simulink library "AtmosphericModel"  (R2024a)
settings: Solver=ode45  StartTime=0.0  StopTime=10.0  RelTol=1e-3  EnableMultiTasking=on
settings Model: Creator=bruno  LastModifiedBy=Caê
settings SolverCC: AlgebraicLoopSolver=TrustRegion
settings DataIOCC: LimitDataPoints=on  ReturnWorkspaceOutputs=off
settings OptimizationCC: LifeSpan=inf
settings DebuggingCC: UnconnectedInputMsg=warning  UnconnectedOutputMsg=warning  UnconnectedLineMsg=warning  AllowSymbolicDim=off  SFUnexpectedBacktrackingDiag=warning  SFNoUnconditionalDefaultTransitionDiag=warning  ArithmeticOperatorsInVariantConditions=warning
settings ModelReferenceCC: EnableRefExpFcnMdlSchedulingChecks=on
settings SFSimCC: SimUseLocalCustomCode=off  CustomCodeUndefinedFunction=UseInterfaceOnly
settings RTWCC: RTWUseLocalCustomCode=off  GPUComputeCapability=3.5
settings CodeAppCC: StateflowObjectComments=on
settings GRTTargetCC: TargetLangStandard=C89/C90 (ANSI)
settings ConfigComp: CovMetricSettings=dw  CovSaveCumulativeToWorkspaceVar=on  CovSaveSingleToWorkspaceVar=on  CovExternalEMLEnable=off

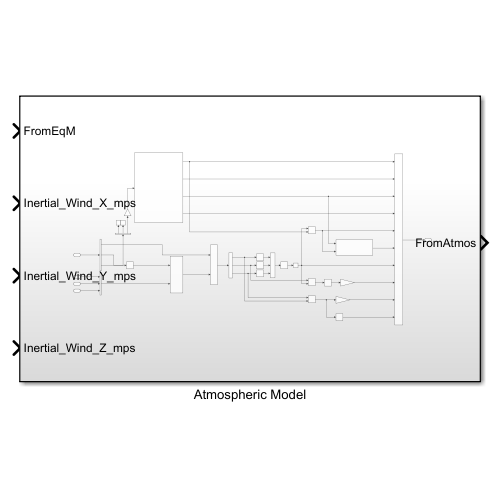
[thumbnail: Simulink's stored preview of the top-level diagram]
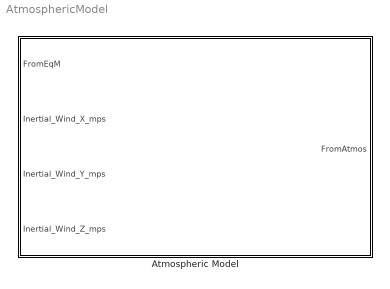
== system AtmosphericModel ==
  Atmospheric Model : Subsystem

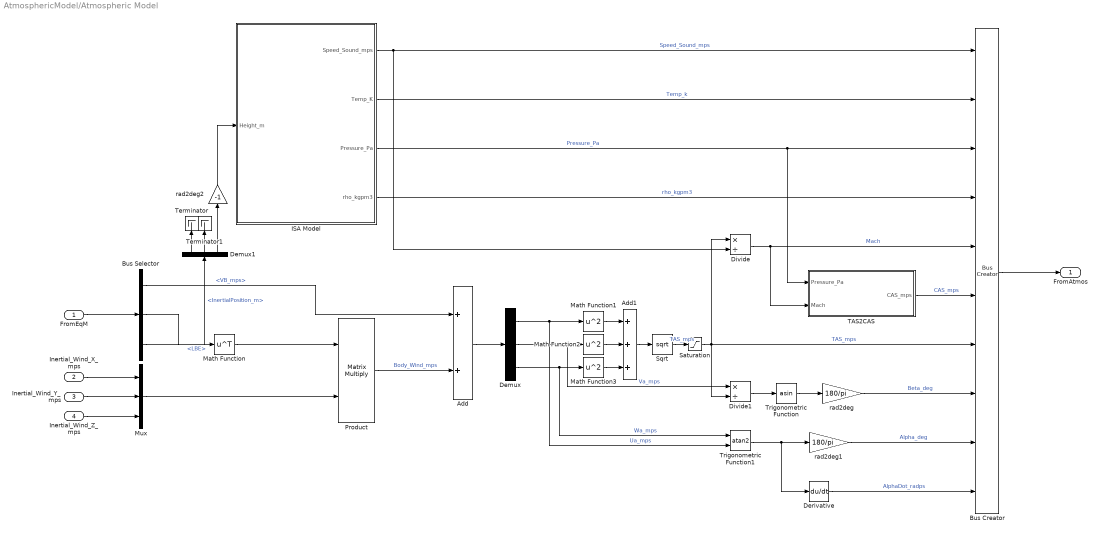
== system AtmosphericModel/Atmospheric Model ==
  FromEqM : Inport
  Inertial_Wind_X_mps : Inport  Port=2
  Inertial_Wind_Y_mps : Inport  Port=3
  Inertial_Wind_Z_mps : Inport  Port=4
  Add : Sum
  Add1 : Sum  Inputs=+++
  Bus Creator : BusCreator  Inputs=10
  Bus Selector : BusSelector  OutputSignals=VB_mps,LBE,InertialPosition_m
  Demux : Demux  Outputs=3
  Demux1 : Demux  Outputs=3
  Derivative : Derivative
  Divide : Product  Inputs=*/
  Divide1 : Product  Inputs=*/
  ISA Model : Subsystem
  Math Function : Math  Operator=transpose  SignedPower=on
  Math Function1 : Math  Operator=square  SignedPower=on
  Math Function2 : Math  Operator=square  SignedPower=on
  Math Function3 : Math  Operator=square  SignedPower=on
  Mux : Mux  Inputs=3
  Product : Product  Multiplication=Matrix(*)
  Saturation : Saturate  UpperLimit=Inf  LowerLimit=0.01
  Sqrt : Sqrt
  TAS2CAS : Subsystem
  Terminator : Terminator
  Terminator1 : Terminator
  Trigonometric Function : Trigonometry  Operator=asin
  Trigonometric Function1 : Trigonometry  Operator=atan2
  rad2deg : Gain  Gain=180/pi
  rad2deg1 : Gain  Gain=180/pi
  rad2deg2 : Gain  Gain=-1
  FromAtmos : Outport
  wires:
  Bus Selector/3 -> Demux1/1  "<InertialPosition_m>"
  Saturation/1 -> Bus Creator/7, Divide1/2, Divide/1  "TAS_mps"
  rad2deg2/1 -> ISA Model/1("Height_m ")
  Demux1/2 -> Terminator1/1
  Demux1/1 -> Terminator/1
  Bus Selector/1 -> Add/1  "<VB_mps>"
  Bus Selector/2 -> Math Function/1  "<LBE>"
  Derivative/1 -> Bus Creator/10  "AlphaDot_radps"
  Trigonometric Function1/1 -> rad2deg1/1, Derivative/1
  Bus Creator/1 -> FromAtmos/1
  rad2deg1/1 -> Bus Creator/9  "Alpha_deg"
  ISA Model/4(rho_kgpm3) -> Bus Creator/4  "rho_kgpm3"
  ISA Model/1(Speed_Sound_mps) -> Divide/2, Bus Creator/1  "Speed_Sound_mps"
  Inertial_Wind_Y_mps/1 -> Mux/2
  ISA Model/2(Temp_K) -> Bus Creator/2  "Temp_k"
  Inertial_Wind_X_mps/1 -> Mux/1
  ISA Model/3(Pressure_Pa) -> Bus Creator/3, TAS2CAS/1(Pressure_Pa)  "Pressure_Pa"
  Divide/1 -> TAS2CAS/2(Mach), Bus Creator/5  "Mach"
  FromEqM/1 -> Bus Selector/1
  Sqrt/1 -> Saturation/1  "TAS_mps"
  Inertial_Wind_Z_mps/1 -> Mux/3
  Math Function/1 -> Product/1
  Mux/1 -> Product/2
  Product/1 -> Add/2  "Body_Wind_mps"
  TAS2CAS/1(CAS_mps) -> Bus Creator/6  "CAS_mps"
  Demux1/3 -> rad2deg2/1
  Add/1 -> Demux/1
  Demux/1 -> Math Function1/1, Trigonometric Function1/2  "Ua_mps"
  Math Function2/1 -> Add1/2
  Trigonometric Function/1 -> rad2deg/1
  Divide1/1 -> Trigonometric Function/1
  Demux/3 -> Math Function3/1, Trigonometric Function1/1  "Wa_mps"
  Demux/2 -> Math Function2/1, Divide1/1  "Va_mps"
  Math Function1/1 -> Add1/1
  Add1/1 -> Sqrt/1
  Math Function3/1 -> Add1/3
  rad2deg/1 -> Bus Creator/8  "Beta_deg"

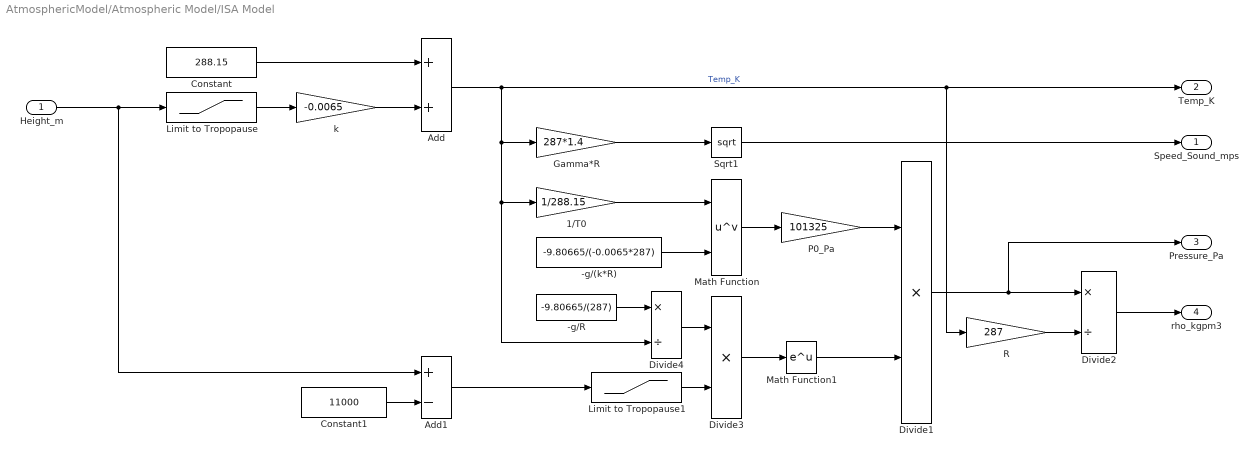
== system AtmosphericModel/Atmospheric Model/ISA Model ==
  "Height_m " : Inport
  -g/(k*R) : Constant  Value=-9.80665/(-0.0065*287)
  -g/R : Constant  Value=-9.80665/(287)
  1/T0 : Gain  Gain=1/288.15
  Add : Sum
  Add1 : Sum  Inputs=+-
  Constant : Constant  Value=288.15
  Constant1 : Constant  Value=11000
  Divide1 : Product  Inputs=**
  Divide2 : Product  Inputs=*/
  Divide3 : Product  Inputs=**
  Divide4 : Product  Inputs=*/
  Gamma*R : Gain  Gain=287*1.4
  Limit to Tropopause : Saturate  UpperLimit=11000  LowerLimit=0
  Limit to Tropopause1 : Saturate  UpperLimit=inf  LowerLimit=0
  Math Function : Math  Operator=pow  SignedPower=on
  Math Function1 : Math  SignedPower=on
  P0_Pa : Gain  Gain=101325
  R : Gain  Gain=287
  Sqrt1 : Sqrt
  k : Gain  Gain=-0.0065
  Speed_Sound_mps : Outport
  Temp_K : Outport  Port=2
  Pressure_Pa : Outport  Port=3
  rho_kgpm3 : Outport  Port=4
  wires:
  Gamma*R/1 -> Sqrt1/1
  Limit to Tropopause/1 -> k/1
  Add/1 -> Divide4/2, 1/T0/1, Gamma*R/1, Temp_K/1, R/1  "Temp_K"
  k/1 -> Add/2
  Constant/1 -> Add/1
  "Height_m "/1 -> Add1/1, Limit to Tropopause/1
  Add1/1 -> Limit to Tropopause1/1
  Limit to Tropopause1/1 -> Divide3/2
  Sqrt1/1 -> Speed_Sound_mps/1
  1/T0/1 -> Math Function/1
  -g/(k*R)/1 -> Math Function/2
  Math Function/1 -> P0_Pa/1
  P0_Pa/1 -> Divide1/1
  Divide1/1 -> Divide2/1, Pressure_Pa/1
  R/1 -> Divide2/2
  Divide2/1 -> rho_kgpm3/1
  Constant1/1 -> Add1/2
  -g/R/1 -> Divide4/1
  Divide4/1 -> Divide3/1
  Divide3/1 -> Math Function1/1
  Math Function1/1 -> Divide1/2

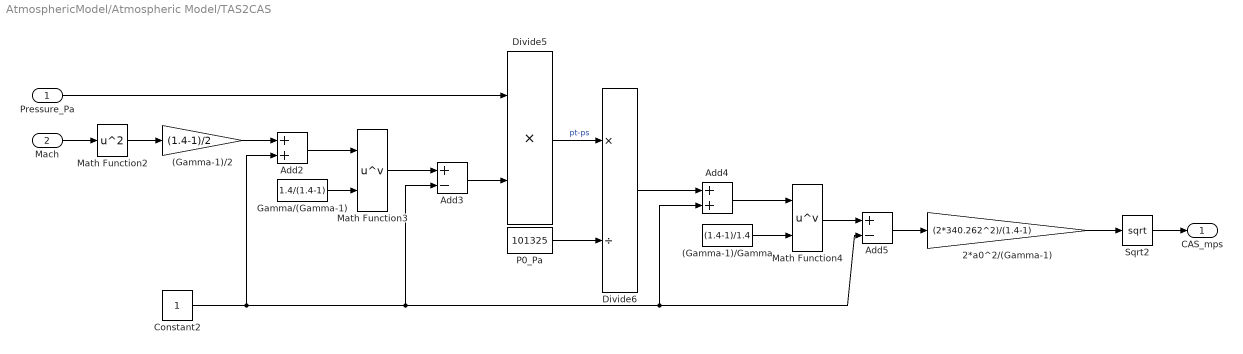
== system AtmosphericModel/Atmospheric Model/TAS2CAS ==
  Pressure_Pa : Inport
  Mach : Inport  Port=2
  (Gamma-1)/2 : Gain  Gain=(1.4-1)/2
  (Gamma-1)/Gamma : Constant  Value=(1.4-1)/1.4
  2*a0^2/(Gamma-1) : Gain  Gain=(2*340.262^2)/(1.4-1)
  Add2 : Sum
  Add3 : Sum  Inputs=+-
  Add4 : Sum
  Add5 : Sum  Inputs=+-
  Constant2 : Constant
  Divide5 : Product  Inputs=**
  Divide6 : Product  Inputs=*/
  Gamma/(Gamma-1) : Constant  Value=1.4/(1.4-1)
  Math Function2 : Math  Operator=square  SignedPower=on
  Math Function3 : Math  Operator=pow  SignedPower=on
  Math Function4 : Math  Operator=pow  SignedPower=on
  P0_Pa : Constant  Value=101325
  Sqrt2 : Sqrt
  CAS_mps : Outport
  wires:
  Math Function2/1 -> (Gamma-1)/2/1
  Mach/1 -> Math Function2/1
  (Gamma-1)/2/1 -> Add2/1
  Constant2/1 -> Add3/2, Add4/2, Add5/2, Add2/2
  Add2/1 -> Math Function3/1
  Gamma/(Gamma-1)/1 -> Math Function3/2
  Add3/1 -> Divide5/2
  Math Function3/1 -> Add3/1
  Pressure_Pa/1 -> Divide5/1
  Divide5/1 -> Divide6/1  "pt-ps"
  P0_Pa/1 -> Divide6/2
  Divide6/1 -> Add4/1
  Add4/1 -> Math Function4/1
  (Gamma-1)/Gamma/1 -> Math Function4/2
  Math Function4/1 -> Add5/1
  Add5/1 -> 2*a0^2/(Gamma-1)/1
  2*a0^2/(Gamma-1)/1 -> Sqrt2/1
  Sqrt2/1 -> CAS_mps/1
